simulink model "Prob3"  (R2020b)
settings: Solver=VariableStepAuto  StartTime=0.0  StopTime=10.0  RelTol=1e-3
settings Model: DataDictionary=Prob3_2005160.sldd  Creator=shoun  LastModifiedBy=shoun

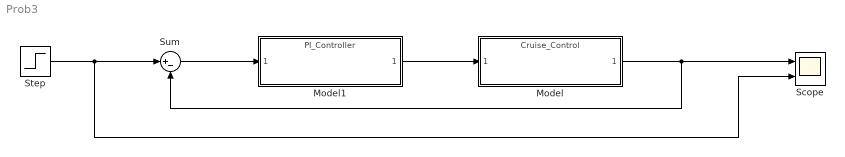
== system Prob3 ==
  Model : ModelReference  ModelNameDialog=Cruise_Control.slx  SimulationMode=Normal  ModelReferenceVersion=1.2
  Model1 : ModelReference  ModelNameDialog=PI_Controller.slx  SimulationMode=Normal  ModelReferenceVersion=1.2
  Scope : Scope  NumInputPorts=2
  Step : Step  SampleTime=0
  Sum : Sum  Inputs=|+-
  wires:
  Step/1 -> Scope/2, Sum/1
  Sum/1 -> Model1/1
  Model1/1 -> Model/1
  Model/1 -> Sum/2, Scope/1
